simulink model "testI2tInputData"  (R2016b)
settings: Solver=FixedStepAuto  StartTime=0.0  StopTime=180  FixedStep=0.002  RelTol=1e-3
libraries: I2t x1
settings Model: Creator=Marc  LastModifiedBy=RKFE
settings DataIOCC: ExternalInput=a  LoadExternalInput=on

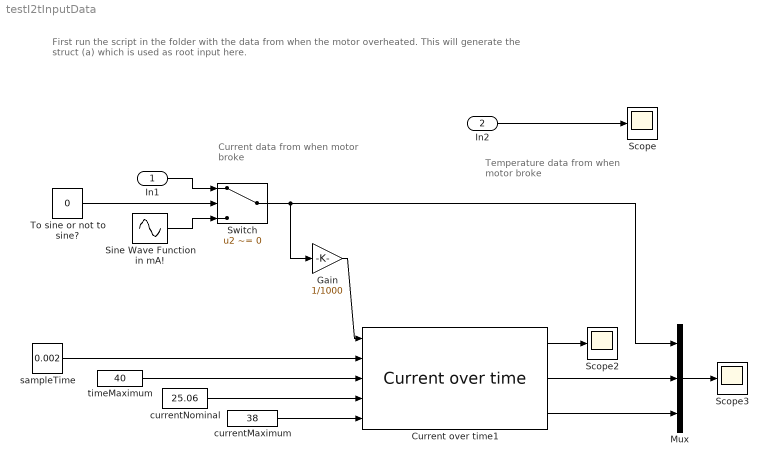
== system testI2tInputData ==
  note: Temperature data from
      | when motor broke
  note: First run the script in the folder with the data from when the motor overheated.
      | This will generate the struct (a) which is used as root input here.
  note: Current data from
      | when motor broke
  In1 : Inport
  In2 : Inport  Port=2
  Current over time1 : I2t/Current over time
  Gain : Gain  Gain=1/1000
  Mux : Mux  Inputs=3
  Scope : Scope
  Scope2 : Scope
  Scope3 : Scope
  Sine Wave Function in mA! : Sin  SineType=Sample based  Amplitude=18000  Bias=20000  Samples=15000  SampleTime=0.002
  Switch : Switch  Criteria=u2 ~= 0
  To sine or not to sine? : Constant  Value=0
  currentMaximum : Constant  Value=38
  currentNominal : Constant  Value=25.06
  sampleTime : Constant  Value=0.002
  timeMaximum : Constant  Value=40
  wires:
  Current over time1/1 -> Scope2/1
  In2/1 -> Scope/1
  In1/1 -> Switch/1
  Mux/1 -> Scope3/1
  Gain/1 -> Current over time1/1
  sampleTime/1 -> Current over time1/2
  Current over time1/2 -> Mux/2
  Current over time1/3 -> Mux/3
  currentNominal/1 -> Current over time1/4
  timeMaximum/1 -> Current over time1/3
  currentMaximum/1 -> Current over time1/5
  Sine Wave Function in mA!/1 -> Switch/3
  Switch/1 -> Mux/1, Gain/1
  To sine or not to sine?/1 -> Switch/2
